simulink model "UnitTestDebug"  (R2018b)
settings: Solver=FixedStepAuto  StartTime=0.0  StopTime=500  FixedStep=fswParams.sample_time_s  RelTol=1e-3
undefined symbols (not defined in the file): DiscIntNeverNeededParam, fswParams, MEKF_lib, simParams, Triad, Triad_lib
libraries: aerolibutil x7, simulink x6, vrlib x4, sharedutil x3, sharedtransform x3, dspmathops x2, satelliteDynamics_lib x1
(part 2 of 2)

== matlab function UnitTestDebug/MATLAB Function1 ==
  data: noise output; u input



function noise   = noise(u)
%         vi=sun_iner;					% stars in the Inertial frame
%          bi=A*vi;							% stars in the Body frame
%  %       sip=bi+randn(3,1)*sigma;sip=sip/norm(sip);	
%  %       stars in the body frame with measeurment error
%  %       Shuster Noise Model, JAS Vol. 38, No. 3, 1990, Eq.(10)
%          z1=(bi(1)/bi(3));z2=(bi(2)/bi(3));
%          rz=sigma^2/(1+z1^2+z2^2)*[(1+z1^2)^2 (z1*z2)^2;(z1*z2)^2 (1+z2^2)^2];
%          [u_z,e_z]=eig(rz);
%          noise1=sqrt(e_z(1,1))*randn(1);noise2=sqrt(e_z(2,2))*randn(1);
%          noise_corr=u_z*[noise1;noise2];
%          alpm=z1+noise_corr(1);betam=z2+noise_corr(2);
%          sip=[alpm;betam;1]/norm([alpm;betam;1]);


x=u(:).'/norm(u);
yz=null(x).';
xyz=[x;yz];
 noise = xyz(2,:)';

         
end

== matlab function UnitTestDebug/MATLAB Function2 ==
  data: noise output; u input



function noise   = noise(u)
%         vi=sun_iner;					% stars in the Inertial frame
%          bi=A*vi;							% stars in the Body frame
%  %       sip=bi+randn(3,1)*sigma;sip=sip/norm(sip);	
%  %       stars in the body frame with measeurment error
%  %       Shuster Noise Model, JAS Vol. 38, No. 3, 1990, Eq.(10)
%          z1=(bi(1)/bi(3));z2=(bi(2)/bi(3));
%          rz=sigma^2/(1+z1^2+z2^2)*[(1+z1^2)^2 (z1*z2)^2;(z1*z2)^2 (1+z2^2)^2];
%          [u_z,e_z]=eig(rz);
%          noise1=sqrt(e_z(1,1))*randn(1);noise2=sqrt(e_z(2,2))*randn(1);
%          noise_corr=u_z*[noise1;noise2];
%          alpm=z1+noise_corr(1);betam=z2+noise_corr(2);
%          sip=[alpm;betam;1]/norm([alpm;betam;1]);


x=u(:).'/norm(u);
yz=null(x).';
xyz=[x;yz];
 noise = xyz(2,:)';

         
end

== matlab function UnitTestDebug/MEKF_lib/Measurement Update/MATLAB Function ==
  data: P_sq output; R_sq input; K output; P_sq input; gyro_valid input; H input
function [P_sq,K] = fcnAQR(R_sq,P_sq, gyro_valid,H)
%#codegen
[nr,~] = size(R_sq);
[np,~] = size(P_sq);
A_QR = [R_sq',zeros(nr,np);(P_sq')*H', P_sq'];

[~,R] = qr(A_QR);
        P_sq = R(7:12,7:12)'; %Updated P_sq
        K_bar = R(1:6,7:12)';    
        Innovation_sq = R(1:6,1:6)';
        
        K = K_bar/(Innovation_sq);
        
        if( gyro_valid == 0 )
    K(4:6,:) = zeros(3,6); %this is done so that we do not update bias based
                            % on false gyro readings
        end
end

== matlab function UnitTestDebug/MEKF_lib/Time Propagation (q,P)/MATLAB Function10 ==
  data: om_mag input; omega_x input; dt input; Phi output
function Phi = Phi_disc(om_mag,omega_x,dt)
%#codegen
% State Transition Matrix
w_n     = om_mag;
w_skew  = omega_x;

if( w_n < 1e-10 )
    Phi = [ eye(3)     -eye(3)*dt;
            zeros(3,3)  eye(3) ];
else
    Phi_11  = eye(3) - w_skew*(sin(w_n*dt)/w_n) + ...
                                        w_skew^2*(1 - cos(w_n*dt))/w_n^2;
    Phi_12  = w_skew*(1 - cos(w_n*dt))/w_n^2 - eye(3)*dt - ...
                                    w_skew^2*(w_n*dt - sin(w_n*dt))/w_n^3;
    Phi_21  = zeros(3,3);    
    Phi_22  = eye(3);    
    Phi     = [ Phi_11 Phi_12;
                Phi_21 Phi_22 ];
end

== matlab function UnitTestDebug/MEKF_lib/Time Propagation (q,P)/MATLAB Function ==
  data: P_sq input; Phi_discrete input; P_sq output; Q_sq input
function P_sq  = Cqr(P_sq,Phi_discrete,Q_sq)
%#codegen

A_QR2 = [P_sq'*Phi_discrete';Q_sq'];
         [~,R2] = qr(A_QR2);
          sq_P_kp1 = R2(1:6,1:6)';
          P_sq = sq_P_kp1;
end

== matlab function UnitTestDebug/MEKF_lib/Measurement Update/P, Kalman Gain ==
  data: R input; Pplus output size=[6,6]; Pminus input; gyro_valid input; H input; K output size=[6,6]
function [Pplus,K] = fcn113(R,Pminus,gyro_valid,H)
K = Pminus*H'/(H*Pminus*H' + R);

if( gyro_valid == 0 )
    K(4:6,:) = zeros(3,6); %this is done so that we do not update bias based
                            % on false gyro readings
end

        KHI = (K*H - eye(6));
        Pplus= KHI*Pminus*KHI' + K*R*K';
end
